simulink model "LiveDisplay"  (R2015b)
settings: Solver=FixedStepDiscrete  StartTime=0.0  StopTime=inf  RelTol=1e-3
StartFcn:
  | PrairieControlSimulink.addEventListenersOnStart
undefined symbols (not defined in the file): pc
libraries: sldrtlib x1
settings Model: Creator=User  LastModifiedBy=User
settings OptimizationCC: BlockReduction=off
settings HardwareCC: ProdBitPerLong=64  ProdLargestAtomicFloat=None  ProdHWDeviceType=Intel->x86-64  TargetBitPerLong=64  TargetBitPerPointer=64  TargetIntDivRoundTo=Zero  TargetEndianess=LittleEndian  TargetWordSize=64  TargetHWDeviceType=Intel->x86-64
settings RTWCC: SystemTargetFile=sldrt.tlc  TemplateMakefile=sldrt.tmf  Description=Simulink Desktop Real-Time  RTWCompilerOptimization=on
settings CodeAppCC: MaxIdLength=95
settings SimulinkDesktopRealTimeCC: TargetPreCompLibLocation=C:\Program Files\MATLAB\R2015b\toolbox\sldrt\lib\win64  TargetLangStandard=C89/C90 (ANSI)  SupportVariableSizeSignals=off

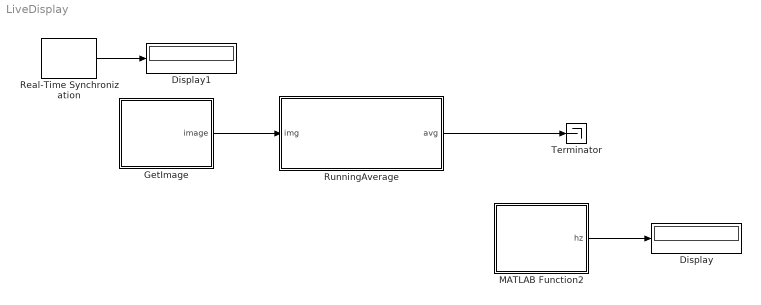
== system LiveDisplay ==
  Display : Display
  Display1 : Display
  GetImage : MATLAB Function  TreatAsAtomicUnit=on  mask{imageSize=pc.getImageMatrixSize}
      mask prompts: imageSize "Image Size"
  MATLAB Function2 : MATLAB Function  TreatAsAtomicUnit=on
  Real-Time Synchronization : sldrtlib/Real-Time Synchronization  SampleTime=1/35  MaxMissedTicks=Inf  ShowMissedTicks=on  YieldWhenWaiting=off
  RunningAverage : MATLAB Function  TreatAsAtomicUnit=on  mask{nFrames=8, outputEvery=16}
      mask prompts: nFrames "Number of Frames"; outputEvery "Output Every"
  Terminator : Terminator
  wires:
  GetImage/1(image) -> RunningAverage/1(img)
  MATLAB Function2/1(hz) -> Display/1
  RunningAverage/1(avg) -> Terminator/1
  Real-Time Synchronization/1 -> Display1/1

== matlab function LiveDisplay/GetImage ==
  data: image output; imageSize parameter size=2
function image = pollImage(imageSize)
%#codegen

image = zeros(imageSize(1), imageSize(2), 'uint16');
coder.extrinsic('pcGetImage');
image = pcGetImage();

== matlab function LiveDisplay/MATLAB Function2 ==
  data: hz output
function hz = getRate()
%#codegen

N = 10;
coder.extrinsic('tic');
coder.extrinsic('toc');
persistent timelog
persistent pos
if isempty(timelog) || isempty(pos)
    timelog = nan(N, 1);
    pos = 1;
    tic;
end


timelog(pos) = toc();
pos = pos + 1;
if pos > N
    pos = 1;
end

mask = ~isnan(timelog);
hz = (nnz(mask)-1) / (max(timelog(mask)) - min(timelog(mask)));

== matlab function LiveDisplay/RunningAverage ==
  data: avg output; img input; nFrames parameter size=1; outputEvery parameter size=1
function avg = runningAverage(img, nFrames, outputEvery)
%#codegen

persistent buffer;
persistent pos;
persistent accum;
assert(nFrames <= 256);

if isempty(buffer) || isempty(pos) || isempty(accum)
    buffer = zeros(size(img, 1), size(img, 2), nFrames, 'uint16');
    pos = 1;
    accum = zeros(size(img, 1), size(img, 2), 'double');
end

accum = accum - double(buffer(:, :, pos));
buffer(:, :, pos) = img;
pos = pos + 1;
if pos > nFrames
    pos = 1;
end

accum = accum + double(img);

avg = accum;
